simulink model "bh_proto_4dof_LAGR_manipulator_CONTROL_DL_and_MOT"  (R2016a)
settings: Solver=ode15s  StartTime=0.0  StopTime=60  FixedStep=0.001  RelTol=1e-5
undefined symbols (not defined in the file or in its folder): b1_damp, b2_damp, b3_damp, b4_damp, g, Hz, L1x, L1y, L1z, L2x, L2y, L2z, L3x, L3y, L3z, mass1, mass2, mass3, mass4, P_mot, Rturn, theta1_0, theta1_dot_0, theta2_0, theta2_dot_0, theta3_0, theta3_dot_0, theta4_0, theta4_dot_0, X, Y, Z
libraries: sm_lib x25, nesl_utility x17, simulink x11, discretizing x2, simulink_extras x2
(part 3 of 3)

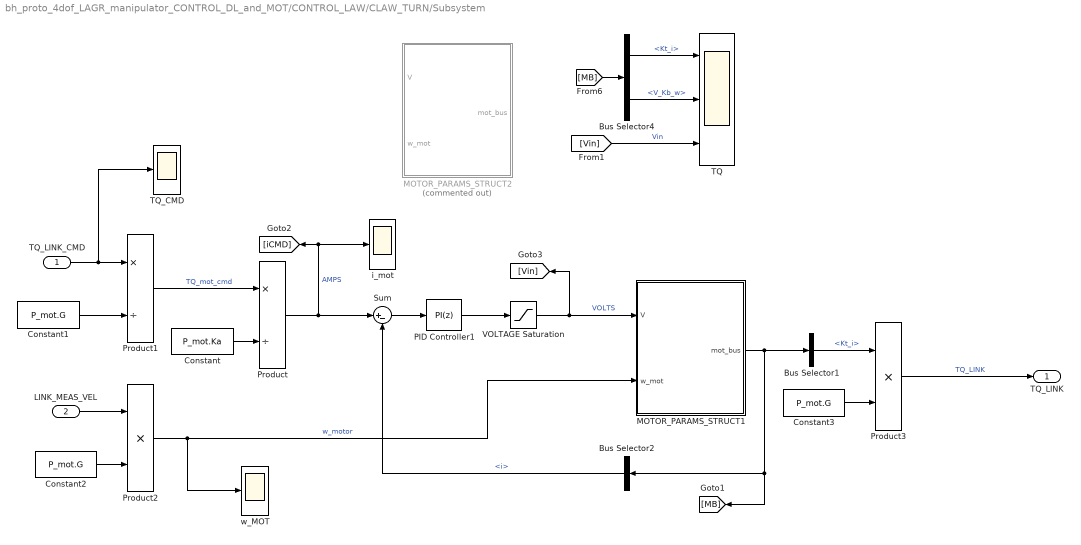
== system bh_proto_4dof_LAGR_manipulator_CONTROL_DL_and_MOT/CONTROL_LAW/CLAW_TURN/Subsystem ==
  TQ_LINK_CMD : Inport
  LINK_MEAS_VEL : Inport  Port=2
  Bus Selector1 : BusSelector  OutputSignals=Kt_i
  Bus Selector2 : BusSelector  OutputSignals=Elec.i
  Bus Selector4 : BusSelector  OutputSignals=Kt_i,Elec.V_Kb_w
  Constant : Constant  Value=P_mot.Ka
  Constant1 : Constant  Value=P_mot.G
  Constant2 : Constant  Value=P_mot.G
  Constant3 : Constant  Value=P_mot.G
  MOTOR_PARAMS_STRUCT1 : Subsystem  mask(DC motor){K=P_mot.Ka, R=P_mot.R, L=P_mot.L, Kb=P_mot.Ke, ID=P_mot.ID}
      mask prompts: K "Torque constant (N.m/A)"; R "Armature resistance (ohms)"; L "Armature Inductance (Henry)"; Kb "Back Emf constant (V.sec/rad)"; ID "Motor_ID  (#1 to #4)"
      mask help: DC motor
      mask Display: disp('DC motor')
  MOTOR_PARAMS_STRUCT2 : Subsystem  Commented=on  mask(DC motor){K=P_mot.Ka, R=P_mot.R, L=P_mot.L, Kb=P_mot.Ke, ID=P_mot.ID}
      mask prompts: K "Torque constant (N.m/A)"; R "Armature resistance (ohms)"; L "Armature Inductance (Henry)"; Kb "Back Emf constant (V.sec/rad)"; ID "Motor_ID  (#1 to #4)"
      mask help: DC motor
      mask Display: disp('DC motor')
  PID Controller1 : simulink/Continuous/PID Controller  Controller=PI  TimeDomain=Discrete-time  SampleTime=0.001  IntegratorMethod=Forward Euler  FilterMethod=Forward Euler  Form=Parallel  UseFilter=on  ControllerParametersSource=internal  P=3.02885793894674  I=6057.71587789348  D=0  N=100  InitialConditionSource=internal  InitialConditionForIntegrator=0  InitialConditionForFilter=0  ExternalReset=none  LimitOutput=off  UpperSaturationLimit=inf  LowerSaturationLimit=-inf  LinearizeAsGain=on  AntiWindupMode=none  Kb=1  TrackingMode=off  Kt=1  PParamMin=[]  PParamMax=[]  IParamMin=[]  IParamMax=[]  DParamMin=[]  DParamMax=[]  NParamMin=[]  NParamMax=[]  KbParamMin=[]  KbParamMax=[]  KtParamMin=[]  KtParamMax=[]  POutMin=[]  POutMax=[]  IOutMin=[]  IOutMax=[]  DOutMin=[]  DOutMax=[]  NOutMin=[]  NOutMax=[]  KbOutMin=[]  KbOutMax=[]  KtOutMin=[]  KtOutMax=[]  IntegratorOutMin=[]  IntegratorOutMax=[]  FilterOutMin=[]  FilterOutMax=[]  SumOutMin=[]  SumOutMax=[]  SumI1OutMin=[]  SumI1OutMax=[]  SumI2OutMin=[]  SumI2OutMax=[]  SumI3OutMin=[]  SumI3OutMax=[]  SumDOutMin=[]  SumDOutMax=[]  SaturationOutMin=[]  SaturationOutMax=[]  IntegratorContinuousStateAttributes=''  IntegratorStateMustResolveToSignalObject=off  IntegratorRTWStateStorageClass=Auto  FilterContinuousStateAttributes=''  FilterStateMustResolveToSignalObject=off  FilterRTWStateStorageClass=Auto  DifferentiatorICPrevScaledInput=0  DifferentiatorOutMin=[]  DifferentiatorOutMax=[]
  Product : Product  Inputs=*/
  Product1 : Product  Inputs=*/
  Product2 : Product
  Product3 : Product
  Sum : Sum  Inputs=|+-
  TQ : Scope  NumInputPorts=3
  TQ_CMD : Scope
  VOLTAGE Saturation : Saturate  UpperLimit=P_mot.Vmax  LowerLimit=-P_mot.Vmax
      settings: AttributesFormatString=|
      | Vmax = %<UpperLimit>
      | Vmin = %<LowerLimit>
  i_mot : Scope
  w_MOT : Scope
  TQ_LINK : Outport
  wires:
  MOTOR_PARAMS_STRUCT1/1(mot_bus) -> Bus Selector1/1, Bus Selector2/1, [MB]
  VOLTAGE Saturation/1 -> MOTOR_PARAMS_STRUCT1/1(V), [Vin]  "VOLTS"
  Product/1 -> Sum/1, i_mot/1, [iCMD]  "AMPS"
  Bus Selector2/1 -> Sum/2  "<i>"
  Sum/1 -> PID Controller1/1
  PID Controller1/1 -> VOLTAGE Saturation/1
  Product2/1 -> MOTOR_PARAMS_STRUCT1/2(w_mot), w_MOT/1  "w_motor"
  [MB] -> Bus Selector4/1
  Bus Selector4/1 -> TQ/1  "<Kt_i>"
  Bus Selector4/2 -> TQ/2  "<V_Kb_w>"
  Constant/1 -> Product/2
  TQ_LINK_CMD/1 -> TQ_CMD/1, Product1/1
  Constant1/1 -> Product1/2
  Product1/1 -> Product/1  "TQ_mot_cmd"
  LINK_MEAS_VEL/1 -> Product2/1
  Constant2/1 -> Product2/2
  Product3/1 -> TQ_LINK/1  "TQ_LINK"
  Bus Selector1/1 -> Product3/1  "<Kt_i>"
  Constant3/1 -> Product3/2
  [Vin] -> TQ/3  "Vin"

== system bh_proto_4dof_LAGR_manipulator_CONTROL_DL_and_MOT/Create_PLANT_BUS/Subsystem1/Subsystem1 ==
  mg_signed : Inport
  Constant : Constant  Value=0
  Mux : Mux  Inputs=3
  Reshape : Reshape  OutputDimensionality=Column vector (2-D)
  COL : Outport
  wires:
  mg_signed/1 -> Mux/3
  Constant/1 -> Mux/2, Mux/1
  Mux/1 -> Reshape/1
  Reshape/1 -> COL/1

== system bh_proto_4dof_LAGR_manipulator_CONTROL_DL_and_MOT/Create_PLANT_BUS/Subsystem1/Subsystem2 ==
  mg_signed : Inport
  Constant : Constant  Value=0
  Mux : Mux  Inputs=3
  Reshape : Reshape  OutputDimensionality=Column vector (2-D)
  COL : Outport
  wires:
  mg_signed/1 -> Mux/3
  Constant/1 -> Mux/2, Mux/1
  Mux/1 -> Reshape/1
  Reshape/1 -> COL/1

== system bh_proto_4dof_LAGR_manipulator_CONTROL_DL_and_MOT/Create_PLANT_BUS/Subsystem1/Subsystem3 ==
  mg_signed : Inport
  Constant : Constant  Value=0
  Mux : Mux  Inputs=3
  Reshape : Reshape  OutputDimensionality=Column vector (2-D)
  COL : Outport
  wires:
  mg_signed/1 -> Mux/3
  Constant/1 -> Mux/2, Mux/1
  Mux/1 -> Reshape/1
  Reshape/1 -> COL/1

== system bh_proto_4dof_LAGR_manipulator_CONTROL_DL_and_MOT/Create_PLANT_BUS/Subsystem1/Subsystem4 ==
  mg_signed : Inport
  Constant : Constant  Value=0
  Mux : Mux  Inputs=3
  Reshape : Reshape  OutputDimensionality=Column vector (2-D)
  COL : Outport
  wires:
  mg_signed/1 -> Mux/3
  Constant/1 -> Mux/2, Mux/1
  Mux/1 -> Reshape/1
  Reshape/1 -> COL/1

== system bh_proto_4dof_LAGR_manipulator_CONTROL_DL_and_MOT/Create_PLANT_BUS/Subsystem1/Subsystem5 ==
  mg_signed : Inport
  Constant : Constant  Value=0
  Mux : Mux  Inputs=3
  Reshape : Reshape  OutputDimensionality=Column vector (2-D)
  COL : Outport
  wires:
  mg_signed/1 -> Mux/3
  Constant/1 -> Mux/2, Mux/1
  Mux/1 -> Reshape/1
  Reshape/1 -> COL/1

== system bh_proto_4dof_LAGR_manipulator_CONTROL_DL_and_MOT/Create_PLANT_BUS/Subsystem1/Subsystem6 ==
  mg_signed : Inport
  Constant : Constant  Value=0
  Mux : Mux  Inputs=3
  Reshape : Reshape  OutputDimensionality=Column vector (2-D)
  COL : Outport
  wires:
  mg_signed/1 -> Mux/3
  Constant/1 -> Mux/2, Mux/1
  Mux/1 -> Reshape/1
  Reshape/1 -> COL/1

== system bh_proto_4dof_LAGR_manipulator_CONTROL_DL_and_MOT/Create_PLANT_BUS1/Subsystem1/Subsystem1 ==
  mg_signed : Inport
  Constant : Constant  Value=0
  Mux : Mux  Inputs=3
  Reshape : Reshape  OutputDimensionality=Column vector (2-D)
  COL : Outport
  wires:
  mg_signed/1 -> Mux/3
  Constant/1 -> Mux/2, Mux/1
  Mux/1 -> Reshape/1
  Reshape/1 -> COL/1

== system bh_proto_4dof_LAGR_manipulator_CONTROL_DL_and_MOT/Create_PLANT_BUS1/Subsystem1/Subsystem2 ==
  mg_signed : Inport
  Constant : Constant  Value=0
  Mux : Mux  Inputs=3
  Reshape : Reshape  OutputDimensionality=Column vector (2-D)
  COL : Outport
  wires:
  mg_signed/1 -> Mux/3
  Constant/1 -> Mux/2, Mux/1
  Mux/1 -> Reshape/1
  Reshape/1 -> COL/1

== system bh_proto_4dof_LAGR_manipulator_CONTROL_DL_and_MOT/Create_PLANT_BUS1/Subsystem1/Subsystem3 ==
  mg_signed : Inport
  Constant : Constant  Value=0
  Mux : Mux  Inputs=3
  Reshape : Reshape  OutputDimensionality=Column vector (2-D)
  COL : Outport
  wires:
  mg_signed/1 -> Mux/3
  Constant/1 -> Mux/2, Mux/1
  Mux/1 -> Reshape/1
  Reshape/1 -> COL/1

== system bh_proto_4dof_LAGR_manipulator_CONTROL_DL_and_MOT/Create_PLANT_BUS1/Subsystem1/Subsystem4 ==
  mg_signed : Inport
  Constant : Constant  Value=0
  Mux : Mux  Inputs=3
  Reshape : Reshape  OutputDimensionality=Column vector (2-D)
  COL : Outport
  wires:
  mg_signed/1 -> Mux/3
  Constant/1 -> Mux/2, Mux/1
  Mux/1 -> Reshape/1
  Reshape/1 -> COL/1

== system bh_proto_4dof_LAGR_manipulator_CONTROL_DL_and_MOT/Create_PLANT_BUS1/Subsystem1/Subsystem5 ==
  mg_signed : Inport
  Constant : Constant  Value=0
  Mux : Mux  Inputs=3
  Reshape : Reshape  OutputDimensionality=Column vector (2-D)
  COL : Outport
  wires:
  mg_signed/1 -> Mux/3
  Constant/1 -> Mux/2, Mux/1
  Mux/1 -> Reshape/1
  Reshape/1 -> COL/1

== system bh_proto_4dof_LAGR_manipulator_CONTROL_DL_and_MOT/Create_PLANT_BUS1/Subsystem1/Subsystem6 ==
  mg_signed : Inport
  Constant : Constant  Value=0
  Mux : Mux  Inputs=3
  Reshape : Reshape  OutputDimensionality=Column vector (2-D)
  COL : Outport
  wires:
  mg_signed/1 -> Mux/3
  Constant/1 -> Mux/2, Mux/1
  Mux/1 -> Reshape/1
  Reshape/1 -> COL/1

== system bh_proto_4dof_LAGR_manipulator_CONTROL_DL_and_MOT/SIMULINK_MODEL/inside_MCKGQ/Subsystem ==
  iTH1 : Inport
  iTH2 : Inport  Port=2
  iTH3 : Inport  Port=3
  iTH4 : Inport  Port=4
  iTH1D : Inport  Port=5
  iTH2D : Inport  Port=6
  iTH3D : Inport  Port=7
  iTH4D : Inport  Port=8
  Bus Creator : BusCreator  Inputs=10
  Bus Selector : BusSelector  OutputSignals=TH1,TH2,TH3,TH4,TH1D,TH2D,TH3D,TH4D
  Mux : Mux
  Mux1 : Mux
  Reshape : Reshape  OutputDimensionality=Column vector (2-D)
  Reshape1 : Reshape  OutputDimensionality=Column vector (2-D)
  Terminator : Terminator
  TH1 : Outport
  TH2 : Outport  Port=2
  TH3 : Outport  Port=3
  TH1D : Outport  Port=4
  TH2D : Outport  Port=5
  TH3D : Outport  Port=6
  TH4D : Outport  Port=7
  TH_BUS : Outport  Port=8
  wires:
  iTH2/1 -> Bus Creator/3, Mux/2  "TH2"
  iTH1/1 -> Bus Creator/2, Mux/1  "TH1"
  iTH2D/1 -> Bus Creator/7, Mux1/2  "TH2D"
  iTH1D/1 -> Bus Creator/6, Mux1/1  "TH1D"
  Mux/1 -> Reshape/1
  Mux1/1 -> Reshape1/1
  Reshape/1 -> Bus Creator/1  "theta_col"
  Reshape1/1 -> Bus Creator/10  "theta_DOT_col"
  Bus Creator/1 -> TH_BUS/1, Bus Selector/1
  iTH3D/1 -> Bus Creator/8, Mux1/3  "TH3D"
  iTH3/1 -> Bus Creator/4, Mux/3  "TH3"
  Bus Selector/1 -> TH1/1  "<TH1>"
  Bus Selector/2 -> TH2/1  "<TH2>"
  Bus Selector/3 -> TH3/1  "<TH3>"
  Bus Selector/5 -> TH1D/1  "<TH1D>"
  Bus Selector/6 -> TH2D/1  "<TH2D>"
  Bus Selector/7 -> TH3D/1  "<TH3D>"
  iTH4/1 -> Bus Creator/5, Mux/4  "TH4"
  iTH4D/1 -> Bus Creator/9, Mux1/4  "TH4D"
  Bus Selector/4 -> Terminator/1  "<TH4>"
  Bus Selector/8 -> TH4D/1  "<TH4D>"

== system bh_proto_4dof_LAGR_manipulator_CONTROL_DL_and_MOT/SIMULINK_MODEL/inside_MCKGQ/Subsystem1 ==
  M : Inport
  C : Inport  Port=2
  K : Inport  Port=3
  G : Inport  Port=4
  Q : Inport  Port=5
  T : Inport  Port=6
  Bus Selector : BusSelector  OutputSignals=theta_DOT_col
  Bus Selector1 : BusSelector  OutputSignals=theta_col
  Demux : Demux
  MATLAB Function : MATLAB Function  TreatAsAtomicUnit=on
  Product : Product  Multiplication=Matrix(*)
  Product1 : Product  Multiplication=Matrix(*)
  Product2 : Product  Inputs=/  Multiplication=Matrix(*)
  Product3 : Product  Multiplication=Matrix(*)
  SC_cond : Scope
  Sum : Sum  Inputs=+|+|+
  Sum1 : Sum  Inputs=|-+
  TH1_DD : Outport
  TH2_DD : Outport  Port=2
  TH3_DD : Outport  Port=3
  TH4_DD : Outport  Port=4
  wires:
  T/1 -> [T]
  C/1 -> Product/1
  [T] -> Bus Selector/1
  Bus Selector/1 -> Product/2  "<theta_DOT_col>"
  K/1 -> Product1/1
  [T] -> Bus Selector1/1
  Bus Selector1/1 -> Product1/2  "<theta_col>"
  Q/1 -> Sum1/2
  Product1/1 -> Sum/2
  G/1 -> Sum/3
  Product/1 -> Sum/1
  Sum/1 -> Sum1/1
  M/1 -> Product2/1, MATLAB Function/1(M)
  Product2/1 -> Product3/1
  Sum1/1 -> Product3/2
  Product3/1 -> Demux/1
  Demux/1 -> TH1_DD/1
  Demux/2 -> TH2_DD/1
  MATLAB Function/1(the_cond) -> SC_cond/1
  Demux/3 -> TH3_DD/1
  Demux/4 -> TH4_DD/1

== system bh_proto_4dof_LAGR_manipulator_CONTROL_DL_and_MOT/CONTROL_LAW/CLAW_LINK1/Subsystem/MOTOR_PARAMS_STRUCT1 ==
  note: Electrical Equation
      | (Kirchoff's Law)
  note: DC Motor - First Principle Equations
  note: L di/dt = V - R i - K_{emf}\fontsize{20}\omega
  V : Inport
  w_mot : Inport  Port=2
  Add : Sum  Inputs=-+-
  Bus Creator2 : BusCreator  Inputs=2
  Bus Creator3 : BusCreator  Inputs=2
  Current : Integrator
  Kemf : Gain  Gain=Kb
  Kt : Gain  Gain=K
  i : Scope
  inductance : Gain  Gain=1/L
  resistance : Gain  Gain=R
  mot_bus : Outport
  wires:
  V/1 -> Add/2
  Bus Creator2/1 -> mot_bus/1
  [V_Kb_w] -> Bus Creator3/1  "V_Kb_w"
  [i] -> Bus Creator3/2  "i"
  Kemf/1 -> Add/1, [V_Kb_w]
  resistance/1 -> Add/3
  Add/1 -> inductance/1
  Current/1 -> i/1, [i], resistance/1, Kt/1  "i"
  inductance/1 -> Current/1  "di/dt"
  Kt/1 -> [TQ_Kt_i]
  Bus Creator3/1 -> Bus Creator2/2  "Elec"
  [TQ_Kt_i] -> Bus Creator2/1  "Kt_i"
  w_mot/1 -> Kemf/1

== system bh_proto_4dof_LAGR_manipulator_CONTROL_DL_and_MOT/CONTROL_LAW/CLAW_LINK1/Subsystem/MOTOR_PARAMS_STRUCT2 ==
  note: Electrical Equation
      | (Kirchoff's Law)
  note: DC Motor - First Principle Equations
  note: V = R i + K_{emf}\fontsize{20}\omega
  V : Inport
  w_mot : Inport  Port=2
  Add : Sum  Inputs=-+
  Bus Creator2 : BusCreator  Inputs=2
  Bus Creator3 : BusCreator  Inputs=2
  Constant : Constant  Value=R
  Kemf : Gain  Gain=Kb
  Kt : Gain  Gain=K
  Product : Product  Inputs=*/
  i : Scope
  mot_bus : Outport
  wires:
  V/1 -> Add/2
  Bus Creator2/1 -> mot_bus/1
  [V_Kb_w] -> Bus Creator3/1  "V_Kb_w"
  [i] -> Bus Creator3/2  "i"
  Kemf/1 -> Add/1, [V_Kb_w]
  Add/1 -> Product/1
  Product/1 -> i/1, [i], Kt/1  "i"
  Kt/1 -> [TQ_Kt_i]
  Bus Creator3/1 -> Bus Creator2/2  "Elec"
  [TQ_Kt_i] -> Bus Creator2/1  "Kt_i"
  w_mot/1 -> Kemf/1
  Constant/1 -> Product/2

== system bh_proto_4dof_LAGR_manipulator_CONTROL_DL_and_MOT/CONTROL_LAW/CLAW_LINK1/Subsystem/MOTOR_PARAMS_STRUCT3 ==
  note: DC Motor - First Principle Equations
  note: L di/dt = V - R i - K_{emf}\fontsize{20}\omega
  note: V = R i + K_{emf}\fontsize{20}\omega
  V : Inport
  w_mot : Inport  Port=2
  Add : Sum  Inputs=-+
  Bus Creator2 : BusCreator  Inputs=2
  Bus Creator3 : BusCreator  Inputs=2
  Kemf : Gain  Gain=Kb
  Kt : Gain  Gain=K
  i : Scope
  resistance : Gain  Gain=1/R
  mot_bus : Outport
  wires:
  V/1 -> Add/2
  Bus Creator2/1 -> mot_bus/1
  [V_Kb_w] -> Bus Creator3/1  "V_Kb_w"
  [i] -> Bus Creator3/2  "i"
  Kemf/1 -> Add/1, [V_Kb_w]
  Add/1 -> resistance/1
  resistance/1 -> i/1, [i], Kt/1  "i"
  Kt/1 -> [TQ_Kt_i]
  Bus Creator3/1 -> Bus Creator2/2  "Elec"
  [TQ_Kt_i] -> Bus Creator2/1  "Kt_i"
  w_mot/1 -> Kemf/1

== system bh_proto_4dof_LAGR_manipulator_CONTROL_DL_and_MOT/CONTROL_LAW/CLAW_TURN/Subsystem/MOTOR_PARAMS_STRUCT1 ==
  note: Electrical Equation
      | (Kirchoff's Law)
  note: DC Motor - First Principle Equations
  note: L di/dt = V - R i - K_{emf}\fontsize{20}\omega
  V : Inport
  w_mot : Inport  Port=2
  Add : Sum  Inputs=-+-
  Bus Creator2 : BusCreator  Inputs=2
  Bus Creator3 : BusCreator  Inputs=2
  Current : Integrator
  Kemf : Gain  Gain=Kb
  Kt : Gain  Gain=K
  i : Scope
  inductance : Gain  Gain=1/L
  resistance : Gain  Gain=R
  mot_bus : Outport
  wires:
  V/1 -> Add/2
  Bus Creator2/1 -> mot_bus/1
  [V_Kb_w] -> Bus Creator3/1  "V_Kb_w"
  [i] -> Bus Creator3/2  "i"
  Kemf/1 -> Add/1, [V_Kb_w]
  resistance/1 -> Add/3
  Add/1 -> inductance/1
  Current/1 -> i/1, [i], resistance/1, Kt/1  "i"
  inductance/1 -> Current/1  "di/dt"
  Kt/1 -> [TQ_Kt_i]
  Bus Creator3/1 -> Bus Creator2/2  "Elec"
  [TQ_Kt_i] -> Bus Creator2/1  "Kt_i"
  w_mot/1 -> Kemf/1

== system bh_proto_4dof_LAGR_manipulator_CONTROL_DL_and_MOT/CONTROL_LAW/CLAW_TURN/Subsystem/MOTOR_PARAMS_STRUCT2 ==
  note: Electrical Equation
      | (Kirchoff's Law)
  note: DC Motor - First Principle Equations
  note: V = R i + K_{emf}\fontsize{20}\omega
  V : Inport
  w_mot : Inport  Port=2
  Add : Sum  Inputs=-+
  Bus Creator2 : BusCreator  Inputs=2
  Bus Creator3 : BusCreator  Inputs=2
  Constant : Constant  Value=R
  Kemf : Gain  Gain=Kb
  Kt : Gain  Gain=K
  Product : Product  Inputs=*/
  i : Scope
  mot_bus : Outport
  wires:
  V/1 -> Add/2
  Bus Creator2/1 -> mot_bus/1
  [V_Kb_w] -> Bus Creator3/1  "V_Kb_w"
  [i] -> Bus Creator3/2  "i"
  Kemf/1 -> Add/1, [V_Kb_w]
  Add/1 -> Product/1
  Product/1 -> i/1, [i], Kt/1  "i"
  Kt/1 -> [TQ_Kt_i]
  Bus Creator3/1 -> Bus Creator2/2  "Elec"
  [TQ_Kt_i] -> Bus Creator2/1  "Kt_i"
  w_mot/1 -> Kemf/1
  Constant/1 -> Product/2

== matlab function bh_proto_4dof_LAGR_manipulator_CONTROL_DL_and_MOT/TRAJECTORY/THE_J ==
  data: L1Y_s input; the_J output; L2Y_s input; L3Y_s input; theta1 input; theta2 input; theta3 input; theta4 input
function the_J = THE_J(L1Y_s,L2Y_s,L3Y_s,theta1,theta2,theta3,theta4)
%#codegen

%    This function was generated by the Symbolic Math Toolbox version 7.0.
%    13-Sep-2016 14:49:06

the_J = reshape([sin(theta4).*(L2Y_s.*sin(theta1+theta2)+L1Y_s.*sin(theta1)+L3Y_s.*sin(theta1+theta2+theta3)),-cos(theta4).*(L2Y_s.*sin(theta1+theta2)+L1Y_s.*sin(theta1)+L3Y_s.*sin(theta1+theta2+theta3)),L2Y_s.*cos(theta1+theta2)+L1Y_s.*cos(theta1)+L3Y_s.*cos(theta1+theta2+theta3),sin(theta4).*(L2Y_s.*sin(theta1+theta2)+L3Y_s.*sin(theta1+theta2+theta3)),-cos(theta4).*(L2Y_s.*sin(theta1+theta2)+L3Y_s.*sin(theta1+theta2+theta3)),L2Y_s.*cos(theta1+theta2)+L3Y_s.*cos(theta1+theta2+theta3),L3Y_s.*sin(theta1+theta2+theta3).*sin(theta4),-L3Y_s.*sin(theta1+theta2+theta3).*cos(theta4),L3Y_s.*cos(theta1+theta2+theta3),-cos(theta4).*(L2Y_s.*cos(theta1+theta2)+L1Y_s.*cos(theta1)+L3Y_s.*cos(theta1+theta2+theta3)),-sin(theta4).*(L2Y_s.*cos(theta1+theta2)+L1Y_s.*cos(theta1)+L3Y_s.*cos(theta1+theta2+theta3)),0.0],[3,4]);

== matlab function bh_proto_4dof_LAGR_manipulator_CONTROL_DL_and_MOT/SIMULINK_MODEL/inside_MCKGQ/MCKGQ ==
  data: L1X_s input; M output; L2X_s input; L3X_s input; L1Y_s input; L2Y_s input; L3Y_s input; L1Z_s input; L2Z_s input; L3Z_s input; R4_s input; TH1_s input; TH2_s input; TH3_s input; TH1_s_D input; TH2_s_D input; TH3_s_D input; TH4_s_D input; b1_s input; b2_s input; b3_s input; b4_s input; g_s input; m1_s input; m2_s input; m3_s input; m4_s input; taum1_s input; taum2_s input; taum3_s input; taum4_s input; C output; K output; G output; Q output
function [M,C,K,G,Q] = MCKGQ(L1X_s,L2X_s,L3X_s,L1Y_s,L2Y_s,L3Y_s,L1Z_s,L2Z_s,L3Z_s,R4_s,TH1_s,TH2_s,TH3_s,TH1_s_D,TH2_s_D,TH3_s_D,TH4_s_D,b1_s,b2_s,b3_s,b4_s,g_s,m1_s,m2_s,m3_s,m4_s,taum1_s,taum2_s,taum3_s,taum4_s)
%#codegen

%    This function was generated by the Symbolic Math Toolbox version 7.0.
%    13-Sep-2016 13:01:16

M = reshape([L1Y_s.^2.*m1_s.*(1.0./3.0)+L1Y_s.^2.*m2_s+L1Y_s.^2.*m3_s+L2Y_s.^2.*m2_s.*(1.0./3.0)+L2Y_s.^2.*m3_s+L3Y_s.^2.*m3_s.*(1.0./3.0)+L1Z_s.^2.*m1_s.*(1.0./1.2e1)+L2Z_s.^2.*m2_s.*(1.0./1.2e1)+L3Z_s.^2.*m3_s.*(1.0./1.2e1)+L1Y_s.*L2Y_s.*m2_s.*cos(TH2_s)+L1Y_s.*L2Y_s.*m3_s.*cos(TH2_s).*2.0+L2Y_s.*L3Y_s.*m3_s.*cos(TH3_s)+L1Y_s.*L3Y_s.*m3_s.*cos(TH2_s+TH3_s),L2Y_s.^2.*m2_s.*(1.0./3.0)+L2Y_s.^2.*m3_s+L3Y_s.^2.*m3_s.*(1.0./3.0)+L2Z_s.^2.*m2_s.*(1.0./1.2e1)+L3Z_s.^2.*m3_s.*(1.0./1.2e1)+L1Y_s.*L2Y_s.*m2_s.*cos(TH2_s).*(1.0./2.0)+L1Y_s.*L2Y_s.*m3_s.*cos(TH2_s)+L2Y_s.*L3Y_s.*m3_s.*cos(TH3_s)+L1Y_s.*L3Y_s.*m3_s.*cos(TH2_s+TH3_s).*(1.0./2.0),m3_s.*(L3Y_s.^2.*4.0+L3Z_s.^2+L1Y_s.*L3Y_s.*cos(TH2_s+TH3_s).*6.0+L2Y_s.*L3Y_s.*cos(TH3_s).*6.0).*(1.0./1.2e1),0.0,L2Y_s.^2.*m2_s.*(1.0./3.0)+L2Y_s.^2.*m3_s+L3Y_s.^2.*m3_s.*(1.0./3.0)+L2Z_s.^2.*m2_s.*(1.0./1.2e1)+L3Z_s.^2.*m3_s.*(1.0./1.2e1)+L1Y_s.*L2Y_s.*m2_s.*cos(TH2_s).*(1.0./2.0)+L1Y_s.*L2Y_s.*m3_s.*cos(TH2_s)+L2Y_s.*L3Y_s.*m3_s.*cos(TH3_s)+L1Y_s.*L3Y_s.*m3_s.*cos(TH2_s+TH3_s).*(1.0./2.0),L2Y_s.^2.*m2_s.*(1.0./3.0)+L2Y_s.^2.*m3_s+L3Y_s.^2.*m3_s.*(1.0./3.0)+L2Z_s.^2.*m2_s.*(1.0./1.2e1)+L3Z_s.^2.*m3_s.*(1.0./1.2e1)+L2Y_s.*L3Y_s.*m3_s.*cos(TH3_s),m3_s.*(L3Y_s.^2.*4.0+L3Z_s.^2+L2Y_s.*L3Y_s.*cos(TH3_s).*6.0).*(1.0./1.2e1),0.0,m3_s.*(L3Y_s.^2.*4.0+L3Z_s.^2+L1Y_s.*L3Y_s.*cos(TH2_s+TH3_s).*6.0+L2Y_s.*L3Y_s.*cos(TH3_s).*6.0).*(1.0./1.2e1),m3_s.*(L3Y_s.^2.*4.0+L3Z_s.^2+L2Y_s.*L3Y_s.*cos(TH3_s).*6.0).*(1.0./1.2e1),m3_s.*(L3Y_s.^2.*4.0+L3Z_s.^2).*(1.0./1.2e1),0.0,0.0,0.0,0.0,L1X_s.^2.*m1_s.*(1.0./1.2e1)+L2X_s.^2.*m2_s.*(1.0./1.2e1)+L3X_s.^2.*m3_s.*(1.0./1.2e1)+L1Y_s.^2.*m1_s.*(1.0./6.0)+L1Y_s.^2.*m2_s.*(1.0./2.0)+L1Y_s.^2.*m3_s.*(1.0./2.0)+L2Y_s.^2.*m2_s.*(1.0./6.0)+L2Y_s.^2.*m3_s.*(1.0./2.0)+L3Y_s.^2.*m3_s.*(1.0./6.0)+L1Z_s.^2.*m1_s.*(1.0./2.4e1)+L2Z_s.^2.*m2_s.*(1.0./2.4e1)+L3Z_s.^2.*m3_s.*(1.0./2.4e1)+R4_s.^2.*m4_s.*(1.0./2.0)+L3Y_s.^2.*m3_s.*cos(TH1_s.*2.0+TH2_s.*2.0+TH3_s.*2.0).*(1.0./6.0)-L3Z_s.^2.*m3_s.*cos(TH1_s.*2.0+TH2_s.*2.0+TH3_s.*2.0).*(1.0./2.4e1)+L1Y_s.^2.*m1_s.*cos(TH1_s.*2.0).*(1.0./6.0)+L1Y_s.^2.*m2_s.*cos(TH1_s.*2.0).*(1.0./2.0)+L1Y_s.^2.*m3_s.*cos(TH1_s.*2.0).*(1.0./2.0)-L1Z_s.^2.*m1_s.*cos(TH1_s.*2.0).*(1.0./2.4e1)+L2Y_s.^2.*m2_s.*cos(TH1_s.*2.0+TH2_s.*2.0).*(1.0./6.0)+L2Y_s.^2.*m3_s.*cos(TH1_s.*2.0+TH2_s.*2.0).*(1.0./2.0)-L2Z_s.^2.*m2_s.*cos(TH1_s.*2.0+TH2_s.*2.0).*(1.0./2.4e1)+L1Y_s.*L2Y_s.*m2_s.*cos(TH2_s).*(1.0./2.0)+L1Y_s.*L2Y_s.*m3_s.*cos(TH2_s)+L2Y_s.*L3Y_s.*m3_s.*cos(TH3_s).*(1.0./2.0)+L1Y_s.*L2Y_s.*m2_s.*cos(TH1_s.*2.0+TH2_s).*(1.0./2.0)+L1Y_s.*L2Y_s.*m3_s.*cos(TH1_s.*2.0+TH2_s)+L1Y_s.*L3Y_s.*m3_s.*cos(TH1_s.*2.0+TH2_s+TH3_s).*(1.0./2.0)+L1Y_s.*L3Y_s.*m3_s.*cos(TH2_s+TH3_s).*(1.0./2.0)+L2Y_s.*L3Y_s.*m3_s.*cos(TH1_s.*2.0+TH2_s.*2.0+TH3_s).*(1.0./2.0)],[4,4]);
if nargout > 1
    C = reshape([-L1Y_s.*L3Y_s.*TH2_s_D.*m3_s.*sin(TH2_s+TH3_s)-L1Y_s.*L3Y_s.*TH3_s_D.*m3_s.*sin(TH2_s+TH3_s)-L1Y_s.*L2Y_s.*TH2_s_D.*m2_s.*sin(TH2_s)-L1Y_s.*L2Y_s.*TH2_s_D.*m3_s.*sin(TH2_s).*2.0-L2Y_s.*L3Y_s.*TH3_s_D.*m3_s.*sin(TH3_s),L1Y_s.*L3Y_s.*TH1_s_D.*m3_s.*sin(TH2_s+TH3_s).*(1.0./2.0)+L1Y_s.*L2Y_s.*TH1_s_D.*m2_s.*sin(TH2_s).*(1.0./2.0)+L1Y_s.*L2Y_s.*TH1_s_D.*m3_s.*sin(TH2_s)-L2Y_s.*L3Y_s.*TH3_s_D.*m3_s.*sin(TH3_s),L3Y_s.*m3_s.*(L1Y_s.*TH1_s_D.*sin(TH2_s+TH3_s)+L2Y_s.*TH1_s_D.*sin(TH3_s)+L2Y_s.*TH2_s_D.*sin(TH3_s).*2.0).*(1.0./2.0),TH4_s_D.*(L3Y_s.^2.*m3_s.*sin(TH1_s.*2.0+TH2_s.*2.0+TH3_s.*2.0).*4.0-L3Z_s.^2.*m3_s.*sin(TH1_s.*2.0+TH2_s.*2.0+TH3_s.*2.0)+L1Y_s.^2.*m1_s.*sin(TH1_s.*2.0).*4.0+L1Y_s.^2.*m2_s.*sin(TH1_s.*2.0).*1.2e1+L1Y_s.^2.*m3_s.*sin(TH1_s.*2.0).*1.2e1-L1Z_s.^2.*m1_s.*sin(TH1_s.*2.0)+L2Y_s.^2.*m2_s.*sin(TH1_s.*2.0+TH2_s.*2.0).*4.0+L2Y_s.^2.*m3_s.*sin(TH1_s.*2.0+TH2_s.*2.0).*1.2e1-L2Z_s.^2.*m2_s.*sin(TH1_s.*2.0+TH2_s.*2.0)+L1Y_s.*L2Y_s.*m2_s.*sin(TH1_s.*2.0+TH2_s).*1.2e1+L1Y_s.*L2Y_s.*m3_s.*sin(TH1_s.*2.0+TH2_s).*2.4e1+L1Y_s.*L3Y_s.*m3_s.*sin(TH1_s.*2.0+TH2_s+TH3_s).*1.2e1+L2Y_s.*L3Y_s.*m3_s.*sin(TH1_s.*2.0+TH2_s.*2.0+TH3_s).*1.2e1).*(-1.0./1.2e1),L1Y_s.*L3Y_s.*TH2_s_D.*m3_s.*sin(TH2_s+TH3_s).*(-1.0./2.0)-L1Y_s.*L3Y_s.*TH3_s_D.*m3_s.*sin(TH2_s+TH3_s)-L1Y_s.*L2Y_s.*TH2_s_D.*m2_s.*sin(TH2_s).*(1.0./2.0)-L1Y_s.*L2Y_s.*TH2_s_D.*m3_s.*sin(TH2_s)-L2Y_s.*L3Y_s.*TH3_s_D.*m3_s.*sin(TH3_s),-L2Y_s.*L3Y_s.*TH3_s_D.*m3_s.*sin(TH3_s),L2Y_s.*L3Y_s.*TH2_s_D.*m3_s.*sin(TH3_s).*(1.0./2.0),TH4_s_D.*(L3Y_s.^2.*m3_s.*sin(TH1_s.*2.0+TH2_s.*2.0+TH3_s.*2.0).*4.0-L3Z_s.^2.*m3_s.*sin(TH1_s.*2.0+TH2_s.*2.0+TH3_s.*2.0)+L2Y_s.^2.*m2_s.*sin(TH1_s.*2.0+TH2_s.*2.0).*4.0+L2Y_s.^2.*m3_s.*sin(TH1_s.*2.0+TH2_s.*2.0).*1.2e1-L2Z_s.^2.*m2_s.*sin(TH1_s.*2.0+TH2_s.*2.0)+L1Y_s.*L2Y_s.*m2_s.*sin(TH2_s).*6.0+L1Y_s.*L2Y_s.*m3_s.*sin(TH2_s).*1.2e1+L1Y_s.*L2Y_s.*m2_s.*sin(TH1_s.*2.0+TH2_s).*6.0+L1Y_s.*L2Y_s.*m3_s.*sin(TH1_s.*2.0+TH2_s).*1.2e1+L1Y_s.*L3Y_s.*m3_s.*sin(TH1_s.*2.0+TH2_s+TH3_s).*6.0+L1Y_s.*L3Y_s.*m3_s.*sin(TH2_s+TH3_s).*6.0+L2Y_s.*L3Y_s.*m3_s.*sin(TH1_s.*2.0+TH2_s.*2.0+TH3_s).*1.2e1).*(-1.0./1.2e1),L3Y_s.*TH3_s_D.*m3_s.*(L1Y_s.*sin(TH2_s+TH3_s)+L2Y_s.*sin(TH3_s)).*(-1.0./2.0),L2Y_s.*L3Y_s.*TH3_s_D.*m3_s.*sin(TH3_s).*(-1.0./2.0),0.0,TH4_s_D.*m3_s.*(L3Y_s.^2.*sin(TH1_s.*2.0+TH2_s.*2.0+TH3_s.*2.0).*4.0-L3Z_s.^2.*sin(TH1_s.*2.0+TH2_s.*2.0+TH3_s.*2.0)+L1Y_s.*L3Y_s.*sin(TH1_s.*2.0+TH2_s+TH3_s).*6.0+L1Y_s.*L3Y_s.*sin(TH2_s+TH3_s).*6.0+L2Y_s.*L3Y_s.*sin(TH1_s.*2.0+TH2_s.*2.0+TH3_s).*6.0+L2Y_s.*L3Y_s.*sin(TH3_s).*6.0).*(-1.0./1.2e1),TH4_s_D.*(L3Y_s.^2.*m3_s.*sin(TH1_s.*2.0+TH2_s.*2.0+TH3_s.*2.0).*4.0-L3Z_s.^2.*m3_s.*sin(TH1_s.*2.0+TH2_s.*2.0+TH3_s.*2.0)+L1Y_s.^2.*m1_s.*sin(TH1_s.*2.0).*4.0+L1Y_s.^2.*m2_s.*sin(TH1_s.*2.0).*1.2e1+L1Y_s.^2.*m3_s.*sin(TH1_s.*2.0).*1.2e1-L1Z_s.^2.*m1_s.*sin(TH1_s.*2.0)+L2Y_s.^2.*m2_s.*sin(TH1_s.*2.0+TH2_s.*2.0).*4.0+L2Y_s.^2.*m3_s.*sin(TH1_s.*2.0+TH2_s.*2.0).*1.2e1-L2Z_s.^2.*m2_s.*sin(TH1_s.*2.0+TH2_s.*2.0)+L1Y_s.*L2Y_s.*m2_s.*sin(TH1_s.*2.0+TH2_s).*1.2e1+L1Y_s.*L2Y_s.*m3_s.*sin(TH1_s.*2.0+TH2_s).*2.4e1+L1Y_s.*L3Y_s.*m3_s.*sin(TH1_s.*2.0+TH2_s+TH3_s).*1.2e1+L2Y_s.*L3Y_s.*m3_s.*sin(TH1_s.*2.0+TH2_s.*2.0+TH3_s).*1.2e1).*(1.0./2.4e1),TH4_s_D.*(L3Y_s.^2.*m3_s.*sin(TH1_s.*2.0+TH2_s.*2.0+TH3_s.*2.0).*4.0-L3Z_s.^2.*m3_s.*sin(TH1_s.*2.0+TH2_s.*2.0+TH3_s.*2.0)+L2Y_s.^2.*m2_s.*sin(TH1_s.*2.0+TH2_s.*2.0).*4.0+L2Y_s.^2.*m3_s.*sin(TH1_s.*2.0+TH2_s.*2.0).*1.2e1-L2Z_s.^2.*m2_s.*sin(TH1_s.*2.0+TH2_s.*2.0)+L1Y_s.*L2Y_s.*m2_s.*sin(TH2_s).*6.0+L1Y_s.*L2Y_s.*m3_s.*sin(TH2_s).*1.2e1+L1Y_s.*L2Y_s.*m2_s.*sin(TH1_s.*2.0+TH2_s).*6.0+L1Y_s.*L2Y_s.*m3_s.*sin(TH1_s.*2.0+TH2_s).*1.2e1+L1Y_s.*L3Y_s.*m3_s.*sin(TH1_s.*2.0+TH2_s+TH3_s).*6.0+L1Y_s.*L3Y_s.*m3_s.*sin(TH2_s+TH3_s).*6.0+L2Y_s.*L3Y_s.*m3_s.*sin(TH1_s.*2.0+TH2_s.*2.0+TH3_s).*1.2e1).*(1.0./2.4e1),TH4_s_D.*m3_s.*(L3Y_s.^2.*sin(TH1_s.*2.0+TH2_s.*2.0+TH3_s.*2.0).*4.0-L3Z_s.^2.*sin(TH1_s.*2.0+TH2_s.*2.0+TH3_s.*2.0)+L1Y_s.*L3Y_s.*sin(TH1_s.*2.0+TH2_s+TH3_s).*6.0+L1Y_s.*L3Y_s.*sin(TH2_s+TH3_s).*6.0+L2Y_s.*L3Y_s.*sin(TH1_s.*2.0+TH2_s.*2.0+TH3_s).*6.0+L2Y_s.*L3Y_s.*sin(TH3_s).*6.0).*(1.0./2.4e1),0.0],[4,4]);
end
if nargout > 2
    K = reshape([0.0,0.0,0.0,0.0,0.0,0.0,0.0,0.0,0.0,0.0,0.0,0.0,0.0,0.0,0.0,0.0],[4,4]);
end
if nargout > 3
    G = [g_s.*(L2Y_s.*m2_s.*cos(TH1_s+TH2_s)+L2Y_s.*m3_s.*cos(TH1_s+TH2_s).*2.0+L1Y_s.*m1_s.*cos(TH1_s)+L1Y_s.*m2_s.*cos(TH1_s).*2.0+L1Y_s.*m3_s.*cos(TH1_s).*2.0+L3Y_s.*m3_s.*cos(TH1_s+TH2_s+TH3_s)).*(1.0./2.0);L3Y_s.*g_s.*m3_s.*cos(TH1_s+TH2_s+TH3_s).*(1.0./2.0)+L2Y_s.*g_s.*m2_s.*cos(TH1_s+TH2_s).*(1.0./2.0)+L2Y_s.*g_s.*m3_s.*cos(TH1_s+TH2_s);L3Y_s.*g_s.*m3_s.*cos(TH1_s+TH2_s+TH3_s).*(1.0./2.0);0.0];
end
if nargout > 4
    Q = [taum1_s-TH1_s_D.*b1_s;taum2_s-TH2_s_D.*b2_s;taum3_s-TH3_s_D.*b3_s;taum4_s-TH4_s_D.*b4_s];
end

== matlab function bh_proto_4dof_LAGR_manipulator_CONTROL_DL_and_MOT/Create_PLANT_BUS1/CALC_BUS/THE_A_EFF_and_O_and_G ==
  data: L1Y_s input; AF_pos_eff output; L2Y_s input; L3Y_s input; theta1 input; theta2 input; theta3 input; AF_pos_O1 output; AF_pos_O2 output; AF_pos_O3 output; AF_pos_G1 output; AF_pos_G2 output; AF_pos_G3 output
function [AF_pos_eff,AF_pos_O1,AF_pos_O2,AF_pos_O3,AF_pos_G1,AF_pos_G2,AF_pos_G3] = THE_A_EFF_and_O_and_G(L1Y_s,L2Y_s,L3Y_s,theta1,theta2,theta3)
%#codegen

%    This function was generated by the Symbolic Math Toolbox version 7.0.
%    15-Sep-2016 15:54:05

AF_pos_eff = [0.0;L2Y_s.*cos(theta1+theta2)+L1Y_s.*cos(theta1)+L3Y_s.*cos(theta1+theta2+theta3);L2Y_s.*sin(theta1+theta2)+L1Y_s.*sin(theta1)+L3Y_s.*sin(theta1+theta2+theta3)];
if nargout > 1
    AF_pos_O1 = [0.0;0.0;0.0];
end
if nargout > 2
    AF_pos_O2 = [0.0;L1Y_s.*cos(theta1);L1Y_s.*sin(theta1)];
end
if nargout > 3
    AF_pos_O3 = [0.0;L2Y_s.*cos(theta1+theta2)+L1Y_s.*cos(theta1);L2Y_s.*sin(theta1+theta2)+L1Y_s.*sin(theta1)];
end
if nargout > 4
    AF_pos_G1 = [0.0;L1Y_s.*cos(theta1).*(1.0./2.0);L1Y_s.*sin(theta1).*(1.0./2.0)];
end
if nargout > 5
    AF_pos_G2 = [0.0;L2Y_s.*cos(theta1+theta2).*(1.0./2.0)+L1Y_s.*cos(theta1);L2Y_s.*sin(theta1+theta2).*(1.0./2.0)+L1Y_s.*sin(theta1)];
end
if nargout > 6
    AF_pos_G3 = [0.0;L2Y_s.*cos(theta1+theta2)+L1Y_s.*cos(theta1)+L3Y_s.*cos(theta1+theta2+theta3).*(1.0./2.0);L2Y_s.*sin(theta1+theta2)+L1Y_s.*sin(theta1)+L3Y_s.*sin(theta1+theta2+theta3).*(1.0./2.0)];
end

== matlab function bh_proto_4dof_LAGR_manipulator_CONTROL_DL_and_MOT/TRAJECTORY/CALC_THETA_DOT ==
  data: J input; TH_DOT output; XY_DOT input; lambda_sq input; alt_TH_DOT output
function [TH_DOT, alt_TH_DOT] = calc_TH_DOT(J, XY_DOT, lambda_sq)
%#codegen

    %% so our problem is this:
    %     J*q_dot = x_dot
    %
    % so a solution is:
    %
    %      q_dot = pinv(J) * x_dot
    
    TH_DOT = pinv(J) * XY_DOT;

    %% we can also penalise the q_dot by applying a weight to it.
    %  this will give us a solution where we get a "smaller" q_dot.  This
    %  acts as a "dampening" agent ... and we notice it most at startup.
    
    % consider solving the REGULARISED problem
    %     [       J_mxn  ] * q_dot =  [ x_dot ]
    %     [lamb^2*I_nxn  ]            [ 0_nx1 ]
    %
    % which we'll wite as:
    %
    %              new_A * q_dot = new_b
    %
    % so a solution is:
    %
    %      q_dot = pinv(new_A) * new_b
    
    [m, n]     = size(J); 
    I_mat      = eye( n ); 
    new_A      = [ J;
                   lambda_sq * I_mat];

    new_b      = [ XY_DOT;
                   zeros(n,1) ];

    alt_TH_DOT = pinv( new_A  ) * new_b;
end

== matlab function bh_proto_4dof_LAGR_manipulator_CONTROL_DL_and_MOT/SIMULINK_MODEL/inside_MCKGQ/Subsystem1/MATLAB Function ==
  data: M input; the_cond output
function the_cond = COND(M)
%#codegen

the_cond = cond(M);

end

== matlab function bh_proto_4dof_LAGR_manipulator_CONTROL_DL_and_MOT/Create_PLANT_BUS1/CALC_BUS/THE_W_EFF_and_O_and_G ==
  data: L1Y_s input; WF_pos_eff output; L2Y_s input; L3Y_s input; theta1 input; theta2 input; theta3 input; theta4 input; WF_pos_O1 output; WF_pos_O2 output; WF_pos_O3 output; WF_pos_G1 output; WF_pos_G2 output; WF_pos_G3 output
function [WF_pos_eff,WF_pos_O1,WF_pos_O2,WF_pos_O3,WF_pos_G1,WF_pos_G2,WF_pos_G3] = THE_W_EFF_and_O_and_G(L1Y_s,L2Y_s,L3Y_s,theta1,theta2,theta3,theta4)
%#codegen

%    This function was generated by the Symbolic Math Toolbox version 7.0.
%    15-Sep-2016 15:32:27

WF_pos_eff = [-sin(theta4).*(L2Y_s.*cos(theta1+theta2)+L1Y_s.*cos(theta1)+L3Y_s.*cos(theta1+theta2+theta3));cos(theta4).*(L2Y_s.*cos(theta1+theta2)+L1Y_s.*cos(theta1)+L3Y_s.*cos(theta1+theta2+theta3));L2Y_s.*sin(theta1+theta2)+L1Y_s.*sin(theta1)+L3Y_s.*sin(theta1+theta2+theta3)];
if nargout > 1
    WF_pos_O1 = [0.0;0.0;0.0];
end
if nargout > 2
    WF_pos_O2 = [-L1Y_s.*cos(theta1).*sin(theta4);L1Y_s.*cos(theta1).*cos(theta4);L1Y_s.*sin(theta1)];
end
if nargout > 3
    WF_pos_O3 = [-sin(theta4).*(L2Y_s.*cos(theta1+theta2)+L1Y_s.*cos(theta1));cos(theta4).*(L2Y_s.*cos(theta1+theta2)+L1Y_s.*cos(theta1));L2Y_s.*sin(theta1+theta2)+L1Y_s.*sin(theta1)];
end
if nargout > 4
    WF_pos_G1 = [L1Y_s.*cos(theta1).*sin(theta4).*(-1.0./2.0);L1Y_s.*cos(theta1).*cos(theta4).*(1.0./2.0);L1Y_s.*sin(theta1).*(1.0./2.0)];
end
if nargout > 5
    WF_pos_G2 = [-sin(theta4).*(L2Y_s.*cos(theta1+theta2).*(1.0./2.0)+L1Y_s.*cos(theta1));cos(theta4).*(L2Y_s.*cos(theta1+theta2).*(1.0./2.0)+L1Y_s.*cos(theta1));L2Y_s.*sin(theta1+theta2).*(1.0./2.0)+L1Y_s.*sin(theta1)];
end
if nargout > 6
    WF_pos_G3 = [-sin(theta4).*(L2Y_s.*cos(theta1+theta2)+L1Y_s.*cos(theta1)+L3Y_s.*cos(theta1+theta2+theta3).*(1.0./2.0));cos(theta4).*(L2Y_s.*cos(theta1+theta2)+L1Y_s.*cos(theta1)+L3Y_s.*cos(theta1+theta2+theta3).*(1.0./2.0));L2Y_s.*sin(theta1+theta2)+L1Y_s.*sin(theta1)+L3Y_s.*sin(theta1+theta2+theta3).*(1.0./2.0)];
end

== matlab function bh_proto_4dof_LAGR_manipulator_CONTROL_DL_and_MOT/Create_PLANT_BUS1/Subsystem1/MATLAB Function ==
  data: r input size=[3 1]; TQ output; F input size=[3 1]
function TQ = CROSS(r,F)
%#codegen

TQ = cross(r,F);

== matlab function bh_proto_4dof_LAGR_manipulator_CONTROL_DL_and_MOT/Create_PLANT_BUS1/Subsystem1/MATLAB Function1 ==
  data: r input size=[3 1]; TQ output; F input size=[3 1]
function TQ = CROSS(r,F)
%#codegen

TQ = cross(r,F);

== matlab function bh_proto_4dof_LAGR_manipulator_CONTROL_DL_and_MOT/Create_PLANT_BUS1/Subsystem1/MATLAB Function2 ==
  data: r input size=[3 1]; TQ output; F input size=[3 1]
function TQ = CROSS(r,F)
%#codegen

TQ = cross(r,F);

== matlab function bh_proto_4dof_LAGR_manipulator_CONTROL_DL_and_MOT/Create_PLANT_BUS1/Subsystem1/MATLAB Function3 ==
  data: r input size=[3 1]; TQ output; F input size=[3 1]
function TQ = CROSS(r,F)
%#codegen

TQ = cross(r,F);

== matlab function bh_proto_4dof_LAGR_manipulator_CONTROL_DL_and_MOT/Create_PLANT_BUS1/Subsystem1/MATLAB Function4 ==
  data: r input size=[3 1]; TQ output; F input size=[3 1]
function TQ = CROSS(r,F)
%#codegen

TQ = cross(r,F);

== matlab function bh_proto_4dof_LAGR_manipulator_CONTROL_DL_and_MOT/Create_PLANT_BUS1/Subsystem1/MATLAB Function5 ==
  data: r input size=[3 1]; TQ output; F input size=[3 1]
function TQ = CROSS(r,F)
%#codegen

TQ = cross(r,F);

== matlab function bh_proto_4dof_LAGR_manipulator_CONTROL_DL_and_MOT/TRAJECTORY/THE_XEYE ==
  data: L1Y_s input; XE output; L2Y_s input; L3Y_s input; theta1 input; theta2 input; theta3 input; theta4 input; YE output; ZE output
function [XE,YE,ZE] = THE_XEYE(L1Y_s,L2Y_s,L3Y_s,theta1,theta2,theta3,theta4)
%#codegen

%    This function was generated by the Symbolic Math Toolbox version 7.0.
%    13-Sep-2016 15:29:58

XE = -sin(theta4).*(L2Y_s.*cos(theta1+theta2)+L1Y_s.*cos(theta1)+L3Y_s.*cos(theta1+theta2+theta3));
if nargout > 1
    YE = cos(theta4).*(L2Y_s.*cos(theta1+theta2)+L1Y_s.*cos(theta1)+L3Y_s.*cos(theta1+theta2+theta3));
end
if nargout > 2
    ZE = L2Y_s.*sin(theta1+theta2)+L1Y_s.*sin(theta1)+L3Y_s.*sin(theta1+theta2+theta3);
end

== matlab function bh_proto_4dof_LAGR_manipulator_CONTROL_DL_and_MOT/Create_PLANT_BUS/CALC_BUS/THE_A_EFF_and_O_and_G ==
  data: L1Y_s input; AF_pos_eff output; L2Y_s input; L3Y_s input; theta1 input; theta2 input; theta3 input; AF_pos_O1 output; AF_pos_O2 output; AF_pos_O3 output; AF_pos_G1 output; AF_pos_G2 output; AF_pos_G3 output
function [AF_pos_eff,AF_pos_O1,AF_pos_O2,AF_pos_O3,AF_pos_G1,AF_pos_G2,AF_pos_G3] = THE_A_EFF_and_O_and_G(L1Y_s,L2Y_s,L3Y_s,theta1,theta2,theta3)
%#codegen

%    This function was generated by the Symbolic Math Toolbox version 7.0.
%    15-Sep-2016 15:54:05

AF_pos_eff = [0.0;L2Y_s.*cos(theta1+theta2)+L1Y_s.*cos(theta1)+L3Y_s.*cos(theta1+theta2+theta3);L2Y_s.*sin(theta1+theta2)+L1Y_s.*sin(theta1)+L3Y_s.*sin(theta1+theta2+theta3)];
if nargout > 1
    AF_pos_O1 = [0.0;0.0;0.0];
end
if nargout > 2
    AF_pos_O2 = [0.0;L1Y_s.*cos(theta1);L1Y_s.*sin(theta1)];
end
if nargout > 3
    AF_pos_O3 = [0.0;L2Y_s.*cos(theta1+theta2)+L1Y_s.*cos(theta1);L2Y_s.*sin(theta1+theta2)+L1Y_s.*sin(theta1)];
end
if nargout > 4
    AF_pos_G1 = [0.0;L1Y_s.*cos(theta1).*(1.0./2.0);L1Y_s.*sin(theta1).*(1.0./2.0)];
end
if nargout > 5
    AF_pos_G2 = [0.0;L2Y_s.*cos(theta1+theta2).*(1.0./2.0)+L1Y_s.*cos(theta1);L2Y_s.*sin(theta1+theta2).*(1.0./2.0)+L1Y_s.*sin(theta1)];
end
if nargout > 6
    AF_pos_G3 = [0.0;L2Y_s.*cos(theta1+theta2)+L1Y_s.*cos(theta1)+L3Y_s.*cos(theta1+theta2+theta3).*(1.0./2.0);L2Y_s.*sin(theta1+theta2)+L1Y_s.*sin(theta1)+L3Y_s.*sin(theta1+theta2+theta3).*(1.0./2.0)];
end

== matlab function bh_proto_4dof_LAGR_manipulator_CONTROL_DL_and_MOT/Create_PLANT_BUS/CALC_BUS/THE_W_EFF_and_O_and_G ==
  data: L1Y_s input; WF_pos_eff output; L2Y_s input; L3Y_s input; theta1 input; theta2 input; theta3 input; theta4 input; WF_pos_O1 output; WF_pos_O2 output; WF_pos_O3 output; WF_pos_G1 output; WF_pos_G2 output; WF_pos_G3 output
function [WF_pos_eff,WF_pos_O1,WF_pos_O2,WF_pos_O3,WF_pos_G1,WF_pos_G2,WF_pos_G3] = THE_W_EFF_and_O_and_G(L1Y_s,L2Y_s,L3Y_s,theta1,theta2,theta3,theta4)
%#codegen

%    This function was generated by the Symbolic Math Toolbox version 7.0.
%    15-Sep-2016 15:32:27

WF_pos_eff = [-sin(theta4).*(L2Y_s.*cos(theta1+theta2)+L1Y_s.*cos(theta1)+L3Y_s.*cos(theta1+theta2+theta3));cos(theta4).*(L2Y_s.*cos(theta1+theta2)+L1Y_s.*cos(theta1)+L3Y_s.*cos(theta1+theta2+theta3));L2Y_s.*sin(theta1+theta2)+L1Y_s.*sin(theta1)+L3Y_s.*sin(theta1+theta2+theta3)];
if nargout > 1
    WF_pos_O1 = [0.0;0.0;0.0];
end
if nargout > 2
    WF_pos_O2 = [-L1Y_s.*cos(theta1).*sin(theta4);L1Y_s.*cos(theta1).*cos(theta4);L1Y_s.*sin(theta1)];
end
if nargout > 3
    WF_pos_O3 = [-sin(theta4).*(L2Y_s.*cos(theta1+theta2)+L1Y_s.*cos(theta1));cos(theta4).*(L2Y_s.*cos(theta1+theta2)+L1Y_s.*cos(theta1));L2Y_s.*sin(theta1+theta2)+L1Y_s.*sin(theta1)];
end
if nargout > 4
    WF_pos_G1 = [L1Y_s.*cos(theta1).*sin(theta4).*(-1.0./2.0);L1Y_s.*cos(theta1).*cos(theta4).*(1.0./2.0);L1Y_s.*sin(theta1).*(1.0./2.0)];
end
if nargout > 5
    WF_pos_G2 = [-sin(theta4).*(L2Y_s.*cos(theta1+theta2).*(1.0./2.0)+L1Y_s.*cos(theta1));cos(theta4).*(L2Y_s.*cos(theta1+theta2).*(1.0./2.0)+L1Y_s.*cos(theta1));L2Y_s.*sin(theta1+theta2).*(1.0./2.0)+L1Y_s.*sin(theta1)];
end
if nargout > 6
    WF_pos_G3 = [-sin(theta4).*(L2Y_s.*cos(theta1+theta2)+L1Y_s.*cos(theta1)+L3Y_s.*cos(theta1+theta2+theta3).*(1.0./2.0));cos(theta4).*(L2Y_s.*cos(theta1+theta2)+L1Y_s.*cos(theta1)+L3Y_s.*cos(theta1+theta2+theta3).*(1.0./2.0));L2Y_s.*sin(theta1+theta2)+L1Y_s.*sin(theta1)+L3Y_s.*sin(theta1+theta2+theta3).*(1.0./2.0)];
end

== matlab function bh_proto_4dof_LAGR_manipulator_CONTROL_DL_and_MOT/Create_PLANT_BUS/Subsystem1/MATLAB Function ==
  data: r input size=[3 1]; TQ output; F input size=[3 1]
function TQ = CROSS(r,F)
%#codegen

TQ = cross(r,F);

== matlab function bh_proto_4dof_LAGR_manipulator_CONTROL_DL_and_MOT/Create_PLANT_BUS/Subsystem1/MATLAB Function1 ==
  data: r input size=[3 1]; TQ output; F input size=[3 1]
function TQ = CROSS(r,F)
%#codegen

TQ = cross(r,F);

== matlab function bh_proto_4dof_LAGR_manipulator_CONTROL_DL_and_MOT/Create_PLANT_BUS/Subsystem1/MATLAB Function2 ==
  data: r input size=[3 1]; TQ output; F input size=[3 1]
function TQ = CROSS(r,F)
%#codegen

TQ = cross(r,F);

== matlab function bh_proto_4dof_LAGR_manipulator_CONTROL_DL_and_MOT/Create_PLANT_BUS/Subsystem1/MATLAB Function3 ==
  data: r input size=[3 1]; TQ output; F input size=[3 1]
function TQ = CROSS(r,F)
%#codegen

TQ = cross(r,F);

== matlab function bh_proto_4dof_LAGR_manipulator_CONTROL_DL_and_MOT/Create_PLANT_BUS/Subsystem1/MATLAB Function4 ==
  data: r input size=[3 1]; TQ output; F input size=[3 1]
function TQ = CROSS(r,F)
%#codegen

TQ = cross(r,F);

== matlab function bh_proto_4dof_LAGR_manipulator_CONTROL_DL_and_MOT/Create_PLANT_BUS/Subsystem1/MATLAB Function5 ==
  data: r input size=[3 1]; TQ output; F input size=[3 1]
function TQ = CROSS(r,F)
%#codegen

TQ = cross(r,F);
